simulink model "SF051A_SnsrOffsLrng"  (R2013b)
settings: Solver=FixedStepDiscrete  SolverMode=SingleTasking  StartTime=0.0  StopTime=1  FixedStep=0.002  RelTol=1e-3
undefined symbols (not defined in the file): ARCHGLBPRM_10MILLISEC_SEC_F32, ARCHGLBPRM_2MILLISEC_SEC_F32, ARCHGLBPRM_2PI_ULS_F32, ARCHGLBPRM_FLOATZEROTHD_ULS_F32, ARCHGLBPRM_PIOVER180_ULS_F32, CNV100MICROSECTOMILLISEC_MILLISECPERCNT_F32, CNV100MICROSECTOSEC_SECPERCNT_F32, COVRAMTRXNIT_ULS_F32, HWAUTHYTHD_ULS_F32, HWTQLRNGSTSLRND_CNT_U08, HWTQLRNGSTSNEGOFFS_CNT_U08, HWTQLRNGSTSNOTLRND_CNT_U08, HWTQLRNGSTSPOSOFFS_CNT_U08, HWTQLRNGSTSZEROOFFS_CNT_U08, HWTQLRNGTMRHILIM_SEC_F32, IDYMTRX_ULS_F32, IVS10MS_ULSPERSEC_F32, LRNGFILTICON_ULS_F32, NvmGetErrSts1, ONE_ULS_F32, SnsrOffsLrnd, SnsrOffsLrngFctEna, SnsrOffsLrngHwAgLrngDrvgDstThd, SnsrOffsLrngHwAgLrngEna, SnsrOffsLrngHwAgLrngHwVelThd, SnsrOffsLrngHwAgLrngSysTqThd, SnsrOffsLrngHwAgLrngSysTqThdMed, SnsrOffsLrngHwAgLrngSysTqThdTrustd, SnsrOffsLrngHwAgLrngSysTqThdWide, SnsrOffsLrngHwAgLrngTi, SnsrOffsLrngHwAgLrngVehSpdThd, SnsrOffsLrngHwAgLrngYawOffsDbnd, SnsrOffsLrngHwAgLrngYawRateThd, SnsrOffsLrngHwAgOffsLim, SnsrOffsLrngHwTqLrngEna, SnsrOffsLrngHwTqLrngEnaTiThd, SnsrOffsLrngHwTqLrngHwAgDbnd, SnsrOffsLrngHwTqLrngHwAgThd, SnsrOffsLrngHwTqLrngHwTqThd, SnsrOffsLrngHwTqLrngHwTqZeroOffsThd, SnsrOffsLrngHwTqLrngHwVelThd, SnsrOffsLrngHwTqLrngMeasTi, SnsrOffsLrngHwTqLrngMeasTiScar, SnsrOffsLrngHwTqLrngSampleImbThd1, SnsrOffsLrngHwTqLrngSampleImbThd2, SnsrOffsLrngHwTqLrngSampleThd1, SnsrOffsLrngHwTqLrngSampleThd2, SnsrOffsLrngHwTqLrngTiWghtCoeff, SnsrOffsLrngHwTqLrngVehSpdThd, SnsrOffsLrngHwTqOffsLim, SnsrOffsLrngSampleCntForHwTqLrngRst, SnsrOffsLrngTqInpDetnPwrEstimnThd, SnsrOffsLrngTqInpDetnSinGenrAmp, SnsrOffsLrngTqInpDetnSinGenrFrq, SnsrOffsLrngTqInpDetnStg1FilGain, SnsrOffsLrngTqInpDetnStg1WinSize, SnsrOffsLrngTqInpDetnStg2FilGainCen, SnsrOffsLrngTqInpDetnStg2FilGainDwn, SnsrOffsLrngTqInpDetnStg2FilGainUp, SnsrOffsLrngTqInpDetnStg2WinSize ... (+15)
libraries: Fil x34, FixdToFloat x17, FloatToFixd x16, NxtrLim x15, simulink x12, NxtrAbslt x12, NxtrNvM x8, NxtrMin x5, NxtrMath x3
(part 8 of 11)

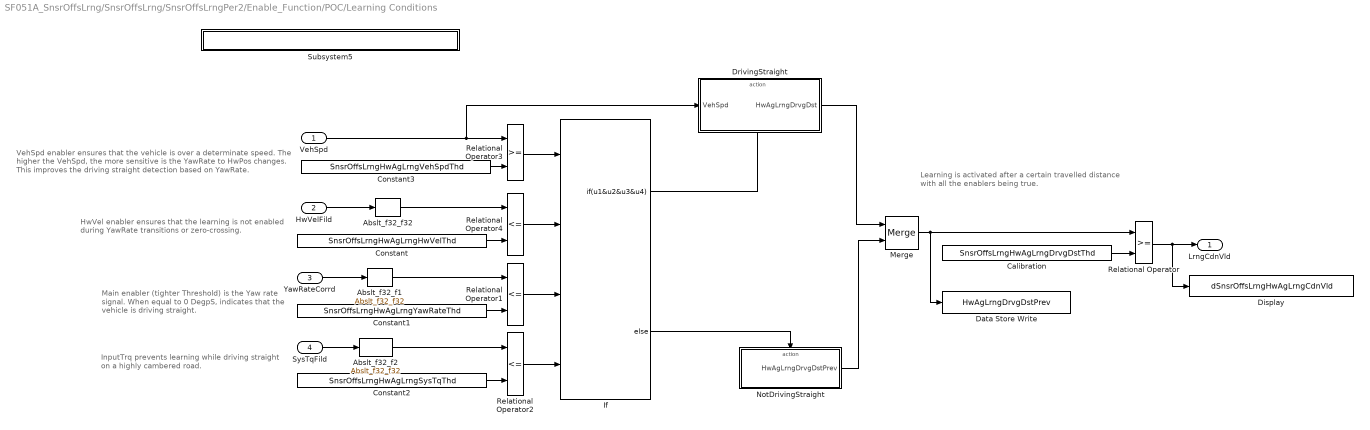
== system SF051A_SnsrOffsLrng/SnsrOffsLrng/SnsrOffsLrngPer2/Enable_Function/POC/Learning Conditions ==
  note: Learning is activated after a certain travelled distance
      |  with all the enablers being true.
  note: InputTrq prevents learning while driving straight
      | on a highly cambered road.
  note: HwVel enabler ensures that the learning is not enabled
      | during YawRate transitions or zero-crossing.
  note: VehSpd enabler ensures that the vehicle is over a determinate speed.
      | The higher the VehSpd, the more sensitive is the YawRate to HwPos
      | changes. This improves the driving straight detection based on YawRate.
  note: Main enabler (tighter Threshold) is the Yaw rate
      | signal. When equal to 0 DegpS, indicates that
      | the vehicle is driving straight.
  VehSpd : Inport  RequirementInfo={'linktype_rmi_doors' '0000babd (/E-STEER Core/SubSystem Specifications/Application Functions/SF051A Sensor Offset Learning)' '#SF051A_125' 'true' 'REQ:SF051A_125' '' } %GIDa_8f59ea37_a6d2_43e8_9752_10147a2ef345
  HwVelFild : Inport  RequirementInfo={'linktype_rmi_doors' '0000babd (/E-STEER Core/SubSystem Specifications/Application Functions/SF051A Sensor Offset Learning)' '#SF051A_125' 'true' 'REQ:SF051A_125' '' } %GIDa_b4c3f45d_537f_4ddb_98c2_1cbec19599c7  Port=2
  YawRateCorrd : Inport  RequirementInfo={'linktype_rmi_doors' '0000babd (/E-STEER Core/SubSystem Specifications/Application Functions/SF051A Sensor Offset Learning)' '#SF051A_125' 'true' 'REQ:SF051A_125' '' } %GIDa_f2d4e035_e9df_4867_bc0f_7342acf6aef2  Port=3
  SysTqFild : Inport  RequirementInfo={'linktype_rmi_doors' '0000babd (/E-STEER Core/SubSystem Specifications/Application Functions/SF051A Sensor Offset Learning)' '#SF051A_125' 'true' 'REQ:SF051A_125' '' } %GIDa_89d517e6_3be2_4d40_b33c_782ff70a0841  Port=4
  Abslt_f32_f1 : NxtrAbslt/Abslt_f32_f32  RequirementInfo={'linktype_rmi_doors' '0000babd (/E-STEER Core/SubSystem Specifications/Application Functions/SF051A Sensor Offset Learning)' '#SF051A_125' 'true' 'REQ:SF051A_125' '' } %GIDa_4a9ff294_23c2_4635_9f2d_79eead891ad6  SFunctionSpec=single y1 = Abslt_f32_f32(single u1)
      settings: AttributesFormatString=%<Name>
  Abslt_f32_f2 : NxtrAbslt/Abslt_f32_f32  RequirementInfo={'linktype_rmi_doors' '0000babd (/E-STEER Core/SubSystem Specifications/Application Functions/SF051A Sensor Offset Learning)' '#SF051A_125' 'true' 'REQ:SF051A_125' '' } %GIDa_bfc6113a_71b3_4014_a79c_4dae946b5258  SFunctionSpec=single y1 = Abslt_f32_f32(single u1)
      settings: AttributesFormatString=%<Name>
  Abslt_f32_f32 : NxtrAbslt/Abslt_f32_f32  RequirementInfo={'linktype_rmi_doors' '0000babd (/E-STEER Core/SubSystem Specifications/Application Functions/SF051A Sensor Offset Learning)' '#SF051A_125' 'true' 'REQ:SF051A_125' '' } %GIDa_d2113858_1e63_4f18_8ebd_0dfc37da8a17  SFunctionSpec=single y1 = Abslt_f32_f32(single u1)
      settings: AttributesFormatString=%<Name>
  Calibration : Constant  RequirementInfo={'linktype_rmi_doors' '0000babd (/E-STEER Core/SubSystem Specifications/Application Functions/SF051A Sensor Offset Learning)' '#SF051A_125' 'true' 'REQ:SF051A_125' '' } %GIDa_a930c023_3647_4bfe_81cc_9ffe63be677e  Value=SnsrOffsLrngHwAgLrngDrvgDstThd  OutDataTypeStr=single
  Constant : Constant  RequirementInfo={'linktype_rmi_doors' '0000babd (/E-STEER Core/SubSystem Specifications/Application Functions/SF051A Sensor Offset Learning)' '#SF051A_125' 'true' 'REQ:SF051A_125' '' } %GIDa_13ca1097_74d2_4314_ac4c_82655165c3ac  Value=SnsrOffsLrngHwAgLrngHwVelThd
  Constant1 : Constant  RequirementInfo={'linktype_rmi_doors' '0000babd (/E-STEER Core/SubSystem Specifications/Application Functions/SF051A Sensor Offset Learning)' '#SF051A_125' 'true' 'REQ:SF051A_125' '' } %GIDa_f59d0f18_d8e0_4a0d_94a2_c992328d5f5a  Value=SnsrOffsLrngHwAgLrngYawRateThd
  Constant2 : Constant  RequirementInfo={'linktype_rmi_doors' '0000babd (/E-STEER Core/SubSystem Specifications/Application Functions/SF051A Sensor Offset Learning)' '#SF051A_125' 'true' 'REQ:SF051A_125' '' } %GIDa_97889c00_0b86_483b_8ac6_8be83d1b4c7e  Value=SnsrOffsLrngHwAgLrngSysTqThd
  Constant3 : Constant  RequirementInfo={'linktype_rmi_doors' '0000babd (/E-STEER Core/SubSystem Specifications/Application Functions/SF051A Sensor Offset Learning)' '#SF051A_125' 'true' 'REQ:SF051A_125' '' } %GIDa_891f1f78_3923_46ac_86af_9c596d3c2421  Value=SnsrOffsLrngHwAgLrngVehSpdThd
  Data Store Write : DataStoreWrite  RequirementInfo={'linktype_rmi_doors' '0000babd (/E-STEER Core/SubSystem Specifications/Application Functions/SF051A Sensor Offset Learning)' '#SF051A_125' 'true' 'REQ:SF051A_125' '' } %GIDa_aa42ae09_446c_4add_b848_b1660a3a4485  DataStoreName=HwAgLrngDrvgDstPrev
  Display : DataStoreWrite  DataStoreName=dSnsrOffsLrngHwAgLrngCdnVld
  DrivingStraight : Subsystem  RequirementInfo={'linktype_rmi_doors' '0000babd (/E-STEER Core/SubSystem Specifications/Application Functions/SF051A Sensor Offset Learning)' '#SF051A_125' 'true' 'REQ:SF051A_125' '' } %GIDa_cc37c45b_3205_4a2a_b2ac_e002ec0e3efb  TreatAsAtomicUnit=on
  If : If  RequirementInfo={'linktype_rmi_doors' '0000babd (/E-STEER Core/SubSystem Specifications/Application Functions/SF051A Sensor Offset Learning)' '#SF051A_125' 'true' 'REQ:SF051A_125' '' } %GIDa_ada5f7e2_fce2_40ad_8932_f71606710b58  NumInputs=4  IfExpression=u1&u2&u3&u4
  Merge : Merge  RequirementInfo={'linktype_rmi_doors' '0000babd (/E-STEER Core/SubSystem Specifications/Application Functions/SF051A Sensor Offset Learning)' '#SF051A_125' 'true' 'REQ:SF051A_125' '' } %GIDa_d84796a1_a26e_43c5_9d0e_55146953274b
  NotDrivingStraight : Subsystem  RequirementInfo={'linktype_rmi_doors' '0000babd (/E-STEER Core/SubSystem Specifications/Application Functions/SF051A Sensor Offset Learning)' '#SF051A_125' 'true' 'REQ:SF051A_125' '' } %GIDa_0603d790_b5f5_4a89_b992_b3578dd6ccf7  TreatAsAtomicUnit=on
  Relational Operator : RelationalOperator  RequirementInfo={'linktype_rmi_doors' '0000babd (/E-STEER Core/SubSystem Specifications/Application Functions/SF051A Sensor Offset Learning)' '#SF051A_125' 'true' 'REQ:SF051A_125' '' } %GIDa_f6c4f543_bc79_4284_beb0_7307c18ad0b4  OutDataTypeStr=boolean
  Relational Operator1 : RelationalOperator  RequirementInfo={'linktype_rmi_doors' '0000babd (/E-STEER Core/SubSystem Specifications/Application Functions/SF051A Sensor Offset Learning)' '#SF051A_125' 'true' 'REQ:SF051A_125' '' } %GIDa_6196e2d7_d842_4412_b387_3769f28bfdab  Operator=<=  OutDataTypeStr=boolean
  Relational Operator2 : RelationalOperator  RequirementInfo={'linktype_rmi_doors' '0000babd (/E-STEER Core/SubSystem Specifications/Application Functions/SF051A Sensor Offset Learning)' '#SF051A_125' 'true' 'REQ:SF051A_125' '' } %GIDa_70a60178_7c67_4179_9a47_94853d13d4d4  Operator=<=  OutDataTypeStr=boolean
  Relational Operator3 : RelationalOperator  RequirementInfo={'linktype_rmi_doors' '0000babd (/E-STEER Core/SubSystem Specifications/Application Functions/SF051A Sensor Offset Learning)' '#SF051A_125' 'true' 'REQ:SF051A_125' '' } %GIDa_022c8ef0_d08f_4bf0_939e_a4515a84757a  OutDataTypeStr=boolean
  Relational Operator4 : RelationalOperator  RequirementInfo={'linktype_rmi_doors' '0000babd (/E-STEER Core/SubSystem Specifications/Application Functions/SF051A Sensor Offset Learning)' '#SF051A_125' 'true' 'REQ:SF051A_125' '' } %GIDa_2be8b1bd_9967_4fbe_97b2_b4364b67bd3a  Operator=<=  OutDataTypeStr=boolean
  Subsystem5 : Subsystem  Description=|  mask(Copyright Information){none=on}
      | Copyright info block.                                               
      |                                                                     
      | Place copyright information at the top of every subsystem in design.
      mask prompts: none "No parameters"
      mask help: Place copyright information at the top of every subsystem in design.
      mask Display:
      | NxtrConf = 'Nexteer Confidential';
      | 
      | sys = bdroot; %handle for the current model ("system")
      | first = get_param(sys,'Created');
      | first = first(end-3:end);  %year is last four digits
      | 
      | last = get_param(sys,'LastModifiedDate');
      | if isempty(last)
      |     last = datestr(now,'yyyy');
      | else
      |     last = last(end-3:end);
      | end
      | 
      | if strcmp(first,last)
      |     fprintf('%s -- Copyright %s Nexteer',NxtrConf,first)
      | else
      |     fprintf('%s -- %s%s- %s Nexteer',NxtrConf,char(169),first,last)
      | end
  LrngCdnVld : Outport
  wires:
  Relational Operator3/1 -> If/1
  HwVelFild/1 -> Abslt_f32_f32/1
  Relational Operator1/1 -> If/3
  Relational Operator4/1 -> If/2
  Abslt_f32_f32/1 -> Relational Operator4/1
  SysTqFild/1 -> Abslt_f32_f2/1
  Relational Operator2/1 -> If/4
  Abslt_f32_f2/1 -> Relational Operator2/1
  Abslt_f32_f1/1 -> Relational Operator1/1
  YawRateCorrd/1 -> Abslt_f32_f1/1
  Constant/1 -> Relational Operator4/2
  Constant1/1 -> Relational Operator1/2
  Constant2/1 -> Relational Operator2/2
  Constant3/1 -> Relational Operator3/2
  If/1 -> DrivingStraight/Action
  If/2 -> NotDrivingStraight/Action
  DrivingStraight/1(HwAgLrngDrvgDst) -> Merge/1
  NotDrivingStraight/1(HwAgLrngDrvgDstPrev) -> Merge/2
  Merge/1 -> Relational Operator/1, Data Store Write/1
  Calibration/1 -> Relational Operator/2
  Relational Operator/1 -> Display/1, LrngCdnVld/1
  VehSpd/1 -> DrivingStraight/1(VehSpd), Relational Operator3/1

== system SF051A_SnsrOffsLrng/SnsrOffsLrng/SnsrOffsLrngPer2/Enable_Function/POC/Reset_HwAg_Learning ==
  note: Suggest coding as inline local function: void Reset_HwAg_Learning()
  note: Set HwAg Offlset learning filter back to the last good learned value written to NVM Ram.
      | Set elapsed learning time back to zero.
  note: Reset timer
  note: Reset filters
  Action Port : ActionPort  ActionType=then
  Constant : Constant  Value=ZERO_ULS_F32  OutDataTypeStr=single
      settings: AttributesFormatString=%<OutDataTypeStr>
  Filter SV : DataStoreWrite  DataStoreName=HwAgLrngFil1  DataStoreElements=HwAgLrngFil1.FilSt
  Filter SV1 : DataStoreWrite  DataStoreName=HwAgLrngFil2  DataStoreElements=HwAgLrngFil2.FilSt
  FixdToFloat_f32_s16 : FixdToFloat/FixdToFloat_f32_s16  Param1=10
  NVMRam_Read : DataStoreRead  DataStoreName=SnsrOffsLrnd  DataStoreElements=SnsrOffsLrnd.YawRateOffs
  Read NVM Ram : DataStoreRead  DataStoreName=SnsrOffsLrnd  DataStoreElements=SnsrOffsLrnd.HwAgOffs
  Subsystem5 : Subsystem  Description=|  mask(Copyright Information){none=on}
      | Copyright info block.                                               
      |                                                                     
      | Place copyright information at the top of every subsystem in design.
      mask prompts: none "No parameters"
      mask help: Place copyright information at the top of every subsystem in design.
      mask Display:
      | NxtrConf = 'Nexteer Confidential';
      | 
      | sys = bdroot; %handle for the current model ("system")
      | first = get_param(sys,'Created');
      | first = first(end-3:end);  %year is last four digits
      | 
      | last = get_param(sys,'LastModifiedDate');
      | if isempty(last)
      |     last = datestr(now,'yyyy');
      | else
      |     last = last(end-3:end);
      | end
      | 
      | if strcmp(first,last)
      |     fprintf('%s -- Copyright %s Nexteer',NxtrConf,first)
      | else
      |     fprintf('%s -- %s%s- %s Nexteer',NxtrConf,char(169),first,last)
      | end
  Update Reference : DataStoreWrite  DataStoreName=SnsrOffsLrnd  DataStoreElements=SnsrOffsLrnd.HwAgLrngYawOffsRef
  Write NVM Ram : DataStoreWrite  DataStoreName=SnsrOffsLrnd  DataStoreElements=SnsrOffsLrnd.HwAgLrndTi
  wires:
  Constant/1 -> Write NVM Ram/1
  Read NVM Ram/1 -> FixdToFloat_f32_s16/1
  NVMRam_Read/1 -> Update Reference/1
  FixdToFloat_f32_s16/1 -> Filter SV1/1, Filter SV/1

== system SF051A_SnsrOffsLrng/SnsrOffsLrng/SnsrOffsLrngPer2/Enable_Function/POC/Subsystem5 ==

== system SF051A_SnsrOffsLrng/SnsrOffsLrng/SnsrOffsLrngPer2/Enable_Function/SOaC_HierarchyManager/POCEnabler ==
  CmnSigVld : Inport  RequirementInfo={'linktype_rmi_doors' '0000babd (/E-STEER Core/SubSystem Specifications/Application Functions/SF051A Sensor Offset Learning)' '#SF051A_135' 'true' 'REQ:SF051A_135' '' } %GIDa_a3a90e4b_a515_4369_8278_0f9e775efabb
  VehYawRateVld : Inport  RequirementInfo={'linktype_rmi_doors' '0000babd (/E-STEER Core/SubSystem Specifications/Application Functions/SF051A Sensor Offset Learning)' '#SF051A_135' 'true' 'REQ:SF051A_135' '' } %GIDa_046d27fa_e356_4762_86a1_0902f3c2ade4  Port=2
  YawRateOffsFrsh : Inport  RequirementInfo={'linktype_rmi_doors' '0000babd (/E-STEER Core/SubSystem Specifications/Application Functions/SF051A Sensor Offset Learning)' '#SF051A_135' 'true' 'REQ:SF051A_135' '' } %GIDa_03f8236f_a4d8_4504_bef2_73d121deb598  Port=3
  Constant1 : Constant  RequirementInfo={'linktype_rmi_doors' '0000babd (/E-STEER Core/SubSystem Specifications/Application Functions/SF051A Sensor Offset Learning)' '#SF051A_136' 'true' 'REQ:SF051A_136' '' ; 'linktype_rmi_doors' '0000babd (/E-STEER Core/SubSystem Specifications/Application Functions/SF051A Sensor Offset Learning)' '#SF051A_135' 'true' 'REQ:SF051A_135' '' } %GIDa_886d2d83_0f18_47ff_afe5_95719c677a16  Value=SnsrOffsLrngHwAgLrngEna
  Display : DataStoreWrite  DataStoreName=dSnsrOffsLrngHwAgLrngEna
  Logical Operator : Logic  RequirementInfo={'linktype_rmi_doors' '0000babd (/E-STEER Core/SubSystem Specifications/Application Functions/SF051A Sensor Offset Learning)' '#SF051A_135' 'true' 'REQ:SF051A_135' '' ; 'linktype_rmi_doors' '0000babd (/E-STEER Core/SubSystem Specifications/Application Functions/SF051A Sensor Offset Learning)' '#SF051A_136' 'true' 'REQ:SF051A_136' '' } %GIDa_e1d92644_86b9_417b_bb7c_d622c0b2c40b  Inputs=5  AllPortsSameDT=off  OutDataTypeStr=boolean
  NvmRam : DataStoreRead  RequirementInfo={'linktype_rmi_doors' '0000babd (/E-STEER Core/SubSystem Specifications/Application Functions/SF051A Sensor Offset Learning)' '#SF051A_135' 'true' 'REQ:SF051A_135' '' } %GIDa_d64055b6_ad18_4625_99bc_bc222697d718  DataStoreName=SnsrOffsLrnd  DataStoreElements=SnsrOffsLrnd.YawRateOffsVld
  Subsystem5 : Subsystem  Description=|  mask(Copyright Information){none=on}
      | Copyright info block.                                               
      |                                                                     
      | Place copyright information at the top of every subsystem in design.
      mask prompts: none "No parameters"
      mask help: Place copyright information at the top of every subsystem in design.
      mask Display:
      | NxtrConf = 'Nexteer Confidential';
      | 
      | sys = bdroot; %handle for the current model ("system")
      | first = get_param(sys,'Created');
      | first = first(end-3:end);  %year is last four digits
      | 
      | last = get_param(sys,'LastModifiedDate');
      | if isempty(last)
      |     last = datestr(now,'yyyy');
      | else
      |     last = last(end-3:end);
      | end
      | 
      | if strcmp(first,last)
      |     fprintf('%s -- Copyright %s Nexteer',NxtrConf,first)
      | else
      |     fprintf('%s -- %s%s- %s Nexteer',NxtrConf,char(169),first,last)
      | end
  HwAgLrngEna : Outport
  wires:
  Logical Operator/1 -> Display/1, HwAgLrngEna/1
  CmnSigVld/1 -> Logical Operator/2
  Constant1/1 -> Logical Operator/1
  YawRateOffsFrsh/1 -> Logical Operator/4
  NvmRam/1 -> Logical Operator/5
  VehYawRateVld/1 -> Logical Operator/3

== system SF051A_SnsrOffsLrng/SnsrOffsLrng/SnsrOffsLrngPer2/Enable_Function/SOaC_HierarchyManager/POCResetLogic ==
  note: Capture the learned Yaw Rate Offset each time that HwAg learning is reset.  If at any time
      | Yaw Rate Offset changes significantly from the captured reference value, reset the HwAg
      | learning routine.  In other words, a major change in Yaw triggers a re-learn of HwAg.
  Abslt_f32_f32 : NxtrAbslt/Abslt_f32_f32  RequirementInfo={'linktype_rmi_doors' '0000babd (/E-STEER Core/SubSystem Specifications/Application Functions/SF051A Sensor Offset Learning)' '#SF051A_134' 'true' 'REQ:SF051A_134' '' } %GIDa_eb268217_533f_429b_abe3_8ca1827af580  SFunctionSpec=single y1 = Abslt_f32_f32(single u1)
      settings: AttributesFormatString=%<Name>
  Constant : Constant  RequirementInfo={'linktype_rmi_doors' '0000babd (/E-STEER Core/SubSystem Specifications/Application Functions/SF051A Sensor Offset Learning)' '#SF051A_134' 'true' 'REQ:SF051A_134' '' } %GIDa_cb9b8ced_48a1_40df_bd9e_7bf129476d0f  Value=SnsrOffsLrngHwAgLrngYawOffsDbnd
  Data Store Read : DataStoreRead  RequirementInfo={'linktype_rmi_doors' '0000babd (/E-STEER Core/SubSystem Specifications/Application Functions/SF051A Sensor Offset Learning)' '#SF051A_134' 'true' 'REQ:SF051A_134' '' } %GIDa_76c40593_7955_4a5c_86c5_bdfe212e95b7  DataStoreName=SnsrOffsLrnd  DataStoreElements=SnsrOffsLrnd.HwAgLrngYawOffsRef
  Display : DataStoreWrite  DataStoreName=dSnsrOffsLrngHwAgLrngRst
  FixdToFloat_f32_s1 : FixdToFloat/FixdToFloat_f32_s16  RequirementInfo={'linktype_rmi_doors' '0000babd (/E-STEER Core/SubSystem Specifications/Application Functions/SF051A Sensor Offset Learning)' '#SF051A_134' 'true' 'REQ:SF051A_134' '' } %GIDa_6455c289_ed33_4177_b6b5_a172c9b77801  Param1=9
  FixdToFloat_f32_s16 : FixdToFloat/FixdToFloat_f32_s16  RequirementInfo={'linktype_rmi_doors' '0000babd (/E-STEER Core/SubSystem Specifications/Application Functions/SF051A Sensor Offset Learning)' '#SF051A_134' 'true' 'REQ:SF051A_134' '' } %GIDa_7b39a599_1da3_484b_8e4f_9eef5a9ab7b8  Param1=9
  NVMRam_Read : DataStoreRead  RequirementInfo={'linktype_rmi_doors' '0000babd (/E-STEER Core/SubSystem Specifications/Application Functions/SF051A Sensor Offset Learning)' '#SF051A_134' 'true' 'REQ:SF051A_134' '' } %GIDa_7759f917_66ca_4690_a4ef_7d43ee1a0bc2  DataStoreName=SnsrOffsLrnd  DataStoreElements=SnsrOffsLrnd.YawRateOffs
  Relational Operator : RelationalOperator  RequirementInfo={'linktype_rmi_doors' '0000babd (/E-STEER Core/SubSystem Specifications/Application Functions/SF051A Sensor Offset Learning)' '#SF051A_134' 'true' 'REQ:SF051A_134' '' } %GIDa_3c7dc04c_6755_4531_889f_25e567f76468  OutDataTypeStr=boolean
  Subsystem5 : Subsystem  Description=|  mask(Copyright Information){none=on}
      | Copyright info block.                                               
      |                                                                     
      | Place copyright information at the top of every subsystem in design.
      mask prompts: none "No parameters"
      mask help: Place copyright information at the top of every subsystem in design.
      mask Display:
      | NxtrConf = 'Nexteer Confidential';
      | 
      | sys = bdroot; %handle for the current model ("system")
      | first = get_param(sys,'Created');
      | first = first(end-3:end);  %year is last four digits
      | 
      | last = get_param(sys,'LastModifiedDate');
      | if isempty(last)
      |     last = datestr(now,'yyyy');
      | else
      |     last = last(end-3:end);
      | end
      | 
      | if strcmp(first,last)
      |     fprintf('%s -- Copyright %s Nexteer',NxtrConf,first)
      | else
      |     fprintf('%s -- %s%s- %s Nexteer',NxtrConf,char(169),first,last)
      | end
  Subtract : Sum  RequirementInfo={'linktype_rmi_doors' '0000babd (/E-STEER Core/SubSystem Specifications/Application Functions/SF051A Sensor Offset Learning)' '#SF051A_134' 'true' 'REQ:SF051A_134' '' } %GIDa_8b9d9596_8162_48c0_9d38_f3b9f3ab54f1  Inputs=+-
  HwAgLrngRst : Outport
  wires:
  Abslt_f32_f32/1 -> Relational Operator/1
  Subtract/1 -> Abslt_f32_f32/1
  Constant/1 -> Relational Operator/2
  NVMRam_Read/1 -> FixdToFloat_f32_s16/1
  Data Store Read/1 -> FixdToFloat_f32_s1/1
  Relational Operator/1 -> Display/1, HwAgLrngRst/1
  FixdToFloat_f32_s16/1 -> Subtract/1
  FixdToFloat_f32_s1/1 -> Subtract/2

== system SF051A_SnsrOffsLrng/SnsrOffsLrng/SnsrOffsLrngPer2/Enable_Function/SOaC_HierarchyManager/Subsystem5 ==

== system SF051A_SnsrOffsLrng/SnsrOffsLrng/SnsrOffsLrngPer2/Enable_Function/SOaC_HierarchyManager/YOCEnabler ==
  note: YOC is enabled if:
      |   - YOCEnable is true
      |   - InputSIgnals Authority is 1
  CmnSigVld : Inport
  VehYawRateVld : Inport  Port=2
  Constant1 : Constant  RequirementInfo={'linktype_rmi_doors' '0000babd (/E-STEER Core/SubSystem Specifications/Application Functions/SF051A Sensor Offset Learning)' '#SF051A_32' 'true' 'REQ:SF051A_32' '' } %GIDa_be471898_d215_4b61_9c96_ada0f6355517  Value=SnsrOffsLrngYawLrngEna
  Display : DataStoreWrite  DataStoreName=dSnsrOffsLrngYawLrngEna
  Logical Operator : Logic  RequirementInfo={'linktype_rmi_doors' '0000babd (/E-STEER Core/SubSystem Specifications/Application Functions/SF051A Sensor Offset Learning)' '#SF051A_32' 'true' 'REQ:SF051A_32' '' } %GIDa_c6731b2d_5e96_4da6_8262_b10b0921fb99  Inputs=3  AllPortsSameDT=off  OutDataTypeStr=boolean
  Subsystem5 : Subsystem  Description=|  mask(Copyright Information){none=on}
      | Copyright info block.                                               
      |                                                                     
      | Place copyright information at the top of every subsystem in design.
      mask prompts: none "No parameters"
      mask help: Place copyright information at the top of every subsystem in design.
      mask Display:
      | NxtrConf = 'Nexteer Confidential';
      | 
      | sys = bdroot; %handle for the current model ("system")
      | first = get_param(sys,'Created');
      | first = first(end-3:end);  %year is last four digits
      | 
      | last = get_param(sys,'LastModifiedDate');
      | if isempty(last)
      |     last = datestr(now,'yyyy');
      | else
      |     last = last(end-3:end);
      | end
      | 
      | if strcmp(first,last)
      |     fprintf('%s -- Copyright %s Nexteer',NxtrConf,first)
      | else
      |     fprintf('%s -- %s%s- %s Nexteer',NxtrConf,char(169),first,last)
      | end
  YawRateLrngEna : Outport
  wires:
  Constant1/1 -> Logical Operator/1
  CmnSigVld/1 -> Logical Operator/2
  Logical Operator/1 -> Display/1, YawRateLrngEna/1
  VehYawRateVld/1 -> Logical Operator/3

== system SF051A_SnsrOffsLrng/SnsrOffsLrng/SnsrOffsLrngPer2/Enable_Function/YOC/Do nothing ==
  Action Port : ActionPort  ActionType=else
  Subsystem5 : Subsystem  Description=|  mask(Copyright Information){none=on}
      | Copyright info block.                                               
      |                                                                     
      | Place copyright information at the top of every subsystem in design.
      mask prompts: none "No parameters"
      mask help: Place copyright information at the top of every subsystem in design.
      mask Display:
      | NxtrConf = 'Nexteer Confidential';
      | 
      | sys = bdroot; %handle for the current model ("system")
      | first = get_param(sys,'Created');
      | first = first(end-3:end);  %year is last four digits
      | 
      | last = get_param(sys,'LastModifiedDate');
      | if isempty(last)
      |     last = datestr(now,'yyyy');
      | else
      |     last = last(end-3:end);
      | end
      | 
      | if strcmp(first,last)
      |     fprintf('%s -- Copyright %s Nexteer',NxtrConf,first)
      | else
      |     fprintf('%s -- %s%s- %s Nexteer',NxtrConf,char(169),first,last)
      | end

== system SF051A_SnsrOffsLrng/SnsrOffsLrng/SnsrOffsLrngPer2/Enable_Function/YOC/Learn ==
  note: Entrance to this subsystem means that vehicle conditions are good for learning.
      |
      | When leaving factory, or after an external reset, consider the learned offset not valid until the filters have had a tunable length of time to
      | attain good approximation of true offset.  Once the learned offset is deemed valid, the timing constraint is removed so that being parked
      | even for a few seconds may tweak the learned value a bit.
      |
      | Filter continuously, but if the duration is not sufficient, do not update NVM RAM with new value.  Next time conditions are good, the filters
      | will continue from their last values.
  note: Filters are continuously active inside this subsystem.  When
      | not in this subystem, the filter state variables are frozen.
  note: Limit changed to a Min block.
  YawRate : Inport
  Action Port : ActionPort  ActionType=then
  Add : Sum  RequirementInfo={'linktype_rmi_doors' '0000babd (/E-STEER Core/SubSystem Specifications/Application Functions/SF051A Sensor Offset Learning)' '#SF051A_90' 'true' 'REQ:SF051A_90' '' } %GIDa_f07b436d_1106_4fd0_930e_f28a3eb3dbeb
  Constant : Constant  RequirementInfo={'linktype_rmi_doors' '0000babd (/E-STEER Core/SubSystem Specifications/Application Functions/SF051A Sensor Offset Learning)' '#SF051A_93' 'true' 'REQ:SF051A_93' '' } %GIDa_394b4221_be42_4a57_8d0b_59a834239b66  Value=SnsrOffsLrngYawLrngTi
  Constant1 : Constant  RequirementInfo={'linktype_rmi_doors' '0000babd (/E-STEER Core/SubSystem Specifications/Application Functions/SF051A Sensor Offset Learning)' '#SF051A_90' 'true' 'REQ:SF051A_90' '' } %GIDa_2c7cd52d_897c_453e_ac97_2e50719e1535  Value=SnsrOffsLrngYawLrngTi
  Constant2 : Constant  RequirementInfo={'linktype_rmi_doors' '0000babd (/E-STEER Core/SubSystem Specifications/Application Functions/SF051A Sensor Offset Learning)' '#SF051A_90' 'true' 'REQ:SF051A_90' '' } %GIDa_9ba959ec_8787_4e5e_bf59_5b49aec7d530  Value=ARCHGLBPRM_10MILLISEC_SEC_F32
  Data Store Read1 : DataStoreRead  RequirementInfo={'linktype_rmi_doors' '0000babd (/E-STEER Core/SubSystem Specifications/Application Functions/SF051A Sensor Offset Learning)' '#SF051A_90' 'true' 'REQ:SF051A_90' '' } %GIDa_8a94f522_706f_4c34_96a1_0958abef325c  DataStoreName=YawLrngElpdLrngTi
  Data Store Read2 : DataStoreRead  RequirementInfo={'linktype_rmi_doors' '0000babd (/E-STEER Core/SubSystem Specifications/Application Functions/SF051A Sensor Offset Learning)' '#SF051A_107' 'true' 'REQ:SF051A_107' '' } %GIDa_e5d570d4_63e2_441f_9653_8a3e1892128d  DataStoreName=SnsrOffsLrnd  DataStoreElements=SnsrOffsLrnd.YawRateOffsVld
  Data Store Write : DataStoreWrite  RequirementInfo={'linktype_rmi_doors' '0000babd (/E-STEER Core/SubSystem Specifications/Application Functions/SF051A Sensor Offset Learning)' '#SF051A_91' 'true' 'REQ:SF051A_91' '' ; 'linktype_rmi_doors' '0000babd (/E-STEER Core/SubSystem Specifications/Application Functions/SF051A Sensor Offset Learning)' '#SF051A_240' 'true' 'REQ:SF051A_240' '' } %GIDa_b4784234_42bd_4e32_bd30_b08c662a4725  DataStoreName=YawLrngElpdLrngTi
  Do nothing : Subsystem  TreatAsAtomicUnit=on
  Filter For Learning : Subsystem
  If : If  RequirementInfo={'linktype_rmi_doors' '0000babd (/E-STEER Core/SubSystem Specifications/Application Functions/SF051A Sensor Offset Learning)' '#SF051A_107' 'true' 'REQ:SF051A_107' '' } %GIDa_5a864c38_8cd9_4e7a_b628_0403566d2c9a  NumInputs=2  IfExpression=u1 | u2
  Min_f32 : NxtrMin/Min_f32  SFunctionSpec=single y1 = Min_f32(single u1, single u2)
      settings: AttributesFormatString=%<Name>
  Relational Operator : RelationalOperator  RequirementInfo={'linktype_rmi_doors' '0000babd (/E-STEER Core/SubSystem Specifications/Application Functions/SF051A Sensor Offset Learning)' '#SF051A_107' 'true' 'REQ:SF051A_107' '' } %GIDa_09260735_486f_484e_9884_e2f31241b5f4  Operator=>  OutDataTypeStr=boolean
  Subsystem5 : Subsystem  Description=|  mask(Copyright Information){none=on}
      | Copyright info block.                                               
      |                                                                     
      | Place copyright information at the top of every subsystem in design.
      mask prompts: none "No parameters"
      mask help: Place copyright information at the top of every subsystem in design.
      mask Display:
      | NxtrConf = 'Nexteer Confidential';
      | 
      | sys = bdroot; %handle for the current model ("system")
      | first = get_param(sys,'Created');
      | first = first(end-3:end);  %year is last four digits
      | 
      | last = get_param(sys,'LastModifiedDate');
      | if isempty(last)
      |     last = datestr(now,'yyyy');
      | else
      |     last = last(end-3:end);
      | end
      | 
      | if strcmp(first,last)
      |     fprintf('%s -- Copyright %s Nexteer',NxtrConf,first)
      | else
      |     fprintf('%s -- %s%s- %s Nexteer',NxtrConf,char(169),first,last)
      | end
  Update NVM RAM : Subsystem  TreatAsAtomicUnit=on
  wires:
  Add/1 -> Min_f32/1, Relational Operator/1  "ElpsdTi_Sec_T_f32"
  YawRate/1 -> Filter For Learning/1(YawRate)
  Filter For Learning/1(LrndBias) -> Update NVM RAM/1(LrndBias)
  If/1 -> Update NVM RAM/Action
  Data Store Read1/1 -> Add/1
  Constant2/1 -> Add/2
  Min_f32/1 -> Data Store Write/1
  Data Store Read2/1 -> If/1
  Constant/1 -> Relational Operator/2
  Relational Operator/1 -> If/2
  If/2 -> Do nothing/Action
  Constant1/1 -> Min_f32/2

== system SF051A_SnsrOffsLrng/SnsrOffsLrng/SnsrOffsLrngPer2/Enable_Function/YOC/Learning Conditions ==
  note: VehSpd = 0 kph is taken as the reference condition
      | for YawRate = 0 DegperS
  note: HwPos <= Threshold is used to prevent learning
      | at very low VehSpd. Vehicle speed sensors are not reliable
      | at values close to 0 kph. If the Hand wheel is in a position near
      | on center, the YawRate signal will not have a big value when the vehicle
      | starts or stops moving.
  note: YawRate <= Threshold  AND YawRate_Gradient <= Threshold
      | are used to prevent learning when the vehicle is located stopped on
      | a moving platform (e.g. Japanish parkings, ferries)
  VehSpd : Inport
  HwAg : Inport  Port=2
  YawA : Inport  Port=3
  YawRateFild : Inport  Port=4  OutDataTypeStr=single
  Abslt_f32_f1 : NxtrAbslt/Abslt_f32_f32  SFunctionSpec=single y1 = Abslt_f32_f32(single u1)
      settings: AttributesFormatString=%<Name>
  Abslt_f32_f2 : NxtrAbslt/Abslt_f32_f32  SFunctionSpec=single y1 = Abslt_f32_f32(single u1)
      settings: AttributesFormatString=%<Name>
  Abslt_f32_f32 : NxtrAbslt/Abslt_f32_f32  SFunctionSpec=single y1 = Abslt_f32_f32(single u1)
      settings: AttributesFormatString=%<Name>
  Add : Sum
  Constant : Constant  Value=SnsrOffsLrngYawLrngHwAgThd
  Constant1 : Constant  Value=SnsrOffsLrngYawLrngYawAThd
  Constant2 : Constant  Value=SnsrOffsLrngYawRateOffsLim
  Constant3 : Constant  Value=YAWRATENOISE_VEHDEGPERSEC_F32
  Display : DataStoreWrite  DataStoreName=dSnsrOffsLrngYawLrngCdnVld
  Float Zero : Constant  Value=ARCHGLBPRM_FLOATZEROTHD_ULS_F32
  Logical Operator : Logic  Inputs=4  AllPortsSameDT=off  OutDataTypeStr=boolean
  Relational Operator{1..4} (4 alike) : RelationalOperator  Operator=<=  OutDataTypeStr=boolean
  Subsystem5 : Subsystem  Description=|  mask(Copyright Information){none=on}
      | Copyright info block.                                               
      |                                                                     
      | Place copyright information at the top of every subsystem in design.
      mask prompts: none "No parameters"
      mask help: Place copyright information at the top of every subsystem in design.
      mask Display:
      | NxtrConf = 'Nexteer Confidential';
      | 
      | sys = bdroot; %handle for the current model ("system")
      | first = get_param(sys,'Created');
      | first = first(end-3:end);  %year is last four digits
      | 
      | last = get_param(sys,'LastModifiedDate');
      | if isempty(last)
      |     last = datestr(now,'yyyy');
      | else
      |     last = last(end-3:end);
      | end
      | 
      | if strcmp(first,last)
      |     fprintf('%s -- Copyright %s Nexteer',NxtrConf,first)
      | else
      |     fprintf('%s -- %s%s- %s Nexteer',NxtrConf,char(169),first,last)
      | end
  LrngCdnVld : Outport
  wires:
  VehSpd/1 -> Relational Operator1/1
  HwAg/1 -> Abslt_f32_f32/1
  Abslt_f32_f32/1 -> Relational Operator4/1
  Relational Operator1/1 -> Logical Operator/1
  Relational Operator4/1 -> Logical Operator/2
  Constant/1 -> Relational Operator4/2
  Float Zero/1 -> Relational Operator1/2
  Abslt_f32_f2/1 -> Relational Operator3/1
  YawA/1 -> Abslt_f32_f2/1
  YawRateFild/1 -> Abslt_f32_f1/1
  Abslt_f32_f1/1 -> Relational Operator2/1
  Constant1/1 -> Relational Operator3/2
  Add/1 -> Relational Operator2/2
  Relational Operator2/1 -> Logical Operator/3
  Relational Operator3/1 -> Logical Operator/4
  Constant3/1 -> Add/1
  Constant2/1 -> Add/2
  Logical Operator/1 -> Display/1, LrngCdnVld/1

== system SF051A_SnsrOffsLrng/SnsrOffsLrng/SnsrOffsLrngPer2/Enable_Function/YOC/Subsystem5 ==

== system SF051A_SnsrOffsLrng/SnsrOffsLrng/SnsrOffsLrngPer1/EnableLearning/EnablingConditions/CheckLastMeasHwPos/FalseOut_KeepRef ==
  Action Port : ActionPort  ActionType=else
  Constant : Constant  Value=false  OutDataTypeStr=boolean
      settings: AttributesFormatString=%<OutDataTypeStr>
  Subsystem5 : Subsystem  Description=|  mask(Copyright Information){none=on}
      | Copyright info block.                                               
      |                                                                     
      | Place copyright information at the top of every subsystem in design.
      mask prompts: none "No parameters"
      mask help: Place copyright information at the top of every subsystem in design.
      mask Display:
      | NxtrConf = 'Nexteer Confidential';
      | 
      | sys = bdroot; %handle for the current model ("system")
      | first = get_param(sys,'Created');
      | first = first(end-3:end);  %year is last four digits
      | 
      | last = get_param(sys,'LastModifiedDate');
      | if isempty(last)
      |     last = datestr(now,'yyyy');
      | else
      |     last = last(end-3:end);
      | end
      | 
      | if strcmp(first,last)
      |     fprintf('%s -- Copyright %s Nexteer',NxtrConf,first)
      | else
      |     fprintf('%s -- %s%s- %s Nexteer',NxtrConf,char(169),first,last)
      | end
  HwAgMoved : Outport
  wires:
  Constant/1 -> HwAgMoved/1

== system SF051A_SnsrOffsLrng/SnsrOffsLrng/SnsrOffsLrngPer1/EnableLearning/EnablingConditions/CheckLastMeasHwPos/Subsystem5 ==

== system SF051A_SnsrOffsLrng/SnsrOffsLrng/SnsrOffsLrngPer1/EnableLearning/EnablingConditions/CheckLastMeasHwPos/TrueOut_ResetRef ==
  Action Port : ActionPort  ActionType=then
  Constant : Constant  Value=true  OutDataTypeStr=boolean
      settings: AttributesFormatString=%<OutDataTypeStr>
  Constant1 : Constant  Value=SYSGLBPRM_HWAGHILIM_HWDEG_F32  OutDataTypeStr=single
  FloatToFixd_s16_f32 : FloatToFixd/FloatToFixd_s16_f32  Param1=4
  NVM write : DataStoreWrite  DataStoreName=SnsrOffsLrnd  DataStoreElements=SnsrOffsLrnd.HwTqLrngHwAgRef
  Subsystem5 : Subsystem  Description=|  mask(Copyright Information){none=on}
      | Copyright info block.                                               
      |                                                                     
      | Place copyright information at the top of every subsystem in design.
      mask prompts: none "No parameters"
      mask help: Place copyright information at the top of every subsystem in design.
      mask Display:
      | NxtrConf = 'Nexteer Confidential';
      | 
      | sys = bdroot; %handle for the current model ("system")
      | first = get_param(sys,'Created');
      | first = first(end-3:end);  %year is last four digits
      | 
      | last = get_param(sys,'LastModifiedDate');
      | if isempty(last)
      |     last = datestr(now,'yyyy');
      | else
      |     last = last(end-3:end);
      | end
      | 
      | if strcmp(first,last)
      |     fprintf('%s -- Copyright %s Nexteer',NxtrConf,first)
      | else
      |     fprintf('%s -- %s%s- %s Nexteer',NxtrConf,char(169),first,last)
      | end
  HwAgMoved : Outport
  wires:
  Constant/1 -> HwAgMoved/1
  Constant1/1 -> FloatToFixd_s16_f32/1
  FloatToFixd_s16_f32/1 -> NVM write/1

== system SF051A_SnsrOffsLrng/SnsrOffsLrng/SnsrOffsLrngPer1/EnableLearning/Eval_Time/GetTiSpan100MicroSec32bit/CopyRight2 ==

== system SF051A_SnsrOffsLrng/SnsrOffsLrng/SnsrOffsLrngPer1/EnableLearning/Eval_Time/GetTiSpan100MicroSec32bit/No wrapping ==
  new : Inport
  ref : Inport  Port=2
  Action Port : ActionPort  ActionType=then
  CopyRight2 : Subsystem  Description=|  mask(Copyright Information){none=on}
      | Copyright info block.                                               
      |                                                                     
      | Place copyright information at the top of every subsystem in design.
      mask prompts: none "No parameters"
      mask help: Place copyright information at the top of every subsystem in design.
      mask Display:
      | NxtrConf = 'Nexteer Confidential';
      | 
      | sys = bdroot; %handle for the current model ("system")
      | first = get_param(sys,'Created');
      | if(isempty(first))
      |     first = datestr(now,'yyyy');
      | else
      |     first = first(end-3:end);  %year is last four digits
      | end
      | 
      | last = get_param(sys,'LastModifiedDate');
      | if isempty(last)
      |     last = datestr(now,'yyyy');
      | else
      |     last = last(end-3:end);
      | end
      | 
      | if strcmp(first,last)
      |     fprintf('%s -- Copyright %s Nexteer',NxtrConf,first)
      | else
      |     fprintf('%s -- %s%s- %s Nexteer',NxtrConf,char(169),first,last)
      | end
  Subtract1 : Sum  Inputs=+-
  Out1 : Outport
  wires:
  ref/1 -> Subtract1/2
  new/1 -> Subtract1/1
  Subtract1/1 -> Out1/1

== system SF051A_SnsrOffsLrng/SnsrOffsLrng/SnsrOffsLrngPer1/EnableLearning/Eval_Time/GetTiSpan100MicroSec32bit/Wrapping ==
  new : Inport
  ref : Inport  Port=2
  Action Port : ActionPort  ActionType=else
  CopyRight2 : Subsystem  Description=|  mask(Copyright Information){none=on}
      | Copyright info block.                                               
      |                                                                     
      | Place copyright information at the top of every subsystem in design.
      mask prompts: none "No parameters"
      mask help: Place copyright information at the top of every subsystem in design.
      mask Display:
      | NxtrConf = 'Nexteer Confidential';
      | 
      | sys = bdroot; %handle for the current model ("system")
      | first = get_param(sys,'Created');
      | if(isempty(first))
      |     first = datestr(now,'yyyy');
      | else
      |     first = first(end-3:end);  %year is last four digits
      | end
      | 
      | last = get_param(sys,'LastModifiedDate');
      | if isempty(last)
      |     last = datestr(now,'yyyy');
      | else
      |     last = last(end-3:end);
      | end
      | 
      | if strcmp(first,last)
      |     fprintf('%s -- Copyright %s Nexteer',NxtrConf,first)
      | else
      |     fprintf('%s -- %s%s- %s Nexteer',NxtrConf,char(169),first,last)
      | end
  Max Counts : Constant  Value=2^32-1  OutDataTypeStr=uint32
  Subtract1 : Sum  Inputs=+-+
  Out1 : Outport
  wires:
  new/1 -> Subtract1/3
  ref/1 -> Subtract1/2
  Max Counts/1 -> Subtract1/1
  Subtract1/1 -> Out1/1

== system SF051A_SnsrOffsLrng/SnsrOffsLrng/SnsrOffsLrngPer1/EnableLearning/False_Reset/GetRefTmr100MicroSec32bit/CopyRight2 ==

== system SF051A_SnsrOffsLrng/SnsrOffsLrng/SnsrOffsLrngPer1/EnableLearning/Perform_TqInpDetn/Do nothing/Subsystem5 ==

== system SF051A_SnsrOffsLrng/SnsrOffsLrng/SnsrOffsLrngPer1/EnableLearning/Perform_TqInpDetn/ElapsedTime/Subsystem5 ==

== system SF051A_SnsrOffsLrng/SnsrOffsLrng/SnsrOffsLrngPer1/EnableLearning/Perform_TqInpDetn/Enable_PreProcessing/False_Hold ==
  Action Port : ActionPort  ActionType=else
  Constant : Constant  Value=false  OutDataTypeStr=boolean
      settings: AttributesFormatString=%<OutDataTypeStr>
  Previous_Value : DataStoreRead  DataStoreName=HwTqLrngTqInpPrsnt
  Subsystem5 : Subsystem  Description=|  mask(Copyright Information){none=on}
      | Copyright info block.                                               
      |                                                                     
      | Place copyright information at the top of every subsystem in design.
      mask prompts: none "No parameters"
      mask help: Place copyright information at the top of every subsystem in design.
      mask Display:
      | NxtrConf = 'Nexteer Confidential';
      | 
      | sys = bdroot; %handle for the current model ("system")
      | first = get_param(sys,'Created');
      | first = first(end-3:end);  %year is last four digits
      | 
      | last = get_param(sys,'LastModifiedDate');
      | if isempty(last)
      |     last = datestr(now,'yyyy');
      | else
      |     last = last(end-3:end);
      | end
      | 
      | if strcmp(first,last)
      |     fprintf('%s -- Copyright %s Nexteer',NxtrConf,first)
      | else
      |     fprintf('%s -- %s%s- %s Nexteer',NxtrConf,char(169),first,last)
      | end
  Vld : Outport
  Prsnt : Outport  Port=2
  wires:
  Constant/1 -> Vld/1
  Previous_Value/1 -> Prsnt/1

== system SF051A_SnsrOffsLrng/SnsrOffsLrng/SnsrOffsLrngPer1/EnableLearning/Perform_TqInpDetn/Enable_PreProcessing/If Action Subsystem ==
  TqInpPrsntRaw : Inport
  Action Port : ActionPort  ActionType=then
  If1 : If  IfExpression=u1
  Merge : Merge
  Merge1 : Merge
  Subsystem5 : Subsystem  Description=|  mask(Copyright Information){none=on}
      | Copyright info block.                                               
      |                                                                     
      | Place copyright information at the top of every subsystem in design.
      mask prompts: none "No parameters"
      mask help: Place copyright information at the top of every subsystem in design.
      mask Display:
      | NxtrConf = 'Nexteer Confidential';
      | 
      | sys = bdroot; %handle for the current model ("system")
      | first = get_param(sys,'Created');
      | first = first(end-3:end);  %year is last four digits
      | 
      | last = get_param(sys,'LastModifiedDate');
      | if isempty(last)
      |     last = datestr(now,'yyyy');
      | else
      |     last = last(end-3:end);
      | end
      | 
      | if strcmp(first,last)
      |     fprintf('%s -- Copyright %s Nexteer',NxtrConf,first)
      | else
      |     fprintf('%s -- %s%s- %s Nexteer',NxtrConf,char(169),first,last)
      | end
  True_False : Subsystem  TreatAsAtomicUnit=on
  True_True : Subsystem  TreatAsAtomicUnit=on
  TqInpPrsntVld : Outport
  TqInpPrsnt : Outport  Port=2
  wires:
  Merge/1 -> TqInpPrsntVld/1
  Merge1/1 -> TqInpPrsnt/1
  True_True/1(Vld) -> Merge/1
  True_False/1(Vld) -> Merge/2
  True_True/2(Prsnt) -> Merge1/1
  True_False/2(Prsnt) -> Merge1/2
  TqInpPrsntRaw/1 -> If1/1
  If1/1 -> True_True/Action
  If1/2 -> True_False/Action

== system SF051A_SnsrOffsLrng/SnsrOffsLrng/SnsrOffsLrngPer1/EnableLearning/Perform_TqInpDetn/Enable_PreProcessing/Preprocessing ==
  note: Runs unconditionally.
  note: Adding two cals at runtime is not efficient, but at
      | least one is likely to be used in online tuning.  Adding
      | them during init would not work for online tuning.
  note: Loop count should = zero when entering this block.
      | Stage 2 block starts execution only after Stage 1 block has been operating for cal1 number of loops.
      | Stage 2 output is only valid once every cal2 number of loops that it has been executing.
  note: Stage 1
  note: Stage 2
  HwTqFild : Inport
  Add : Sum
  Constant : Constant  Value=SnsrOffsLrngTqInpDetnStg1WinSize
  Constant1 : Constant  Value=SnsrOffsLrngTqInpDetnStg2WinSize
  Data Store Write : DataStoreWrite  DataStoreName=TqInpDetnHwTqPreProc
  Data Type Conversion1 : DataTypeConversion  OutDataTypeStr=uint16
  Display1 : DataStoreWrite  DataStoreName=dSnsrOffsLrngTqInpDetnStg1Outp
  Do nothing : Subsystem  TreatAsAtomicUnit=on
  General_Goertzel : Subsystem  TreatAsAtomicUnit=on
  If : If  IfExpression=u1
  If1 : If  IfExpression=u1
  Merge : Merge
  NewOut_ResetCntr : Subsystem  TreatAsAtomicUnit=on
  PrevOut_NoReset : Subsystem  TreatAsAtomicUnit=on
  Relational Operator : RelationalOperator  OutDataTypeStr=boolean
  Relational Operator1 : RelationalOperator  Operator=<  OutDataTypeStr=boolean
  SampleCounter : Subsystem
  Sliding_Goertzel_ver001 : Subsystem
  Subsystem5 : Subsystem  Description=|  mask(Copyright Information){none=on}
      | Copyright info block.                                               
      |                                                                     
      | Place copyright information at the top of every subsystem in design.
      mask prompts: none "No parameters"
      mask help: Place copyright information at the top of every subsystem in design.
      mask Display:
      | NxtrConf = 'Nexteer Confidential';
      | 
      | sys = bdroot; %handle for the current model ("system")
      | first = get_param(sys,'Created');
      | first = first(end-3:end);  %year is last four digits
      | 
      | last = get_param(sys,'LastModifiedDate');
      | if isempty(last)
      |     last = datestr(now,'yyyy');
      | else
      |     last = last(end-3:end);
      | end
      | 
      | if strcmp(first,last)
      |     fprintf('%s -- Copyright %s Nexteer',NxtrConf,first)
      | else
      |     fprintf('%s -- %s%s- %s Nexteer',NxtrConf,char(169),first,last)
      | end
  SampleCntrLim : Outport
  HwTrqPreproc : Outport  Port=2
  wires:
  Sliding_Goertzel_ver001/1(Stg1Outp) -> Display1/1, General_Goertzel/1(Stg1Outp)  "Stg1Outp"
  HwTqFild/1 -> Sliding_Goertzel_ver001/1(HwTqFild)
  If/1 -> General_Goertzel/Action
  General_Goertzel/1(FrqDwnS0) -> NewOut_ResetCntr/1(FrqDwnS0)
  SampleCounter/1(TqInpDetnPreProcEnaLoop) -> Relational Operator/1, [ProcEna], Relational Operator1/1
  Constant1/1 -> Add/1
  If1/2 -> NewOut_ResetCntr/Action
  If1/1 -> PrevOut_NoReset/Action
  PrevOut_NoReset/1(HwTqPreproc) -> Merge/1
  NewOut_ResetCntr/1(HwTqPreproc) -> Merge/2
  Merge/1 -> HwTrqPreproc/1, Data Store Write/1
  General_Goertzel/4(FrqCenS1) -> NewOut_ResetCntr/4(FrqCenS1)
  General_Goertzel/3(FrqCenS0) -> NewOut_ResetCntr/3(FrqCenS0)
  General_Goertzel/6(FrqUpS1) -> NewOut_ResetCntr/6(FrqUpS1)
  General_Goertzel/5(FrqUpS0) -> NewOut_ResetCntr/5(FrqUpS0)
  General_Goertzel/2(FrqDwnS1) -> NewOut_ResetCntr/2(FrqDwnS1)
  Constant/1 -> Data Type Conversion1/1
  Data Type Conversion1/1 -> Relational Operator/2, Add/2
  Add/1 -> SampleCounter/1(HiLim), [CntrLim], SampleCntrLim/1
  Relational Operator/1 -> If/1
  Relational Operator1/1 -> If1/1
  [CntrLim] -> Relational Operator1/2
  If/2 -> Do nothing/Action
  [ProcEna] -> PrevOut_NoReset/1(TqInpDetnPreProcEnaLoop)

== system SF051A_SnsrOffsLrng/SnsrOffsLrng/SnsrOffsLrngPer1/EnableLearning/Perform_TqInpDetn/Enable_PreProcessing/Subsystem5 ==

== system SF051A_SnsrOffsLrng/SnsrOffsLrng/SnsrOffsLrngPer1/EnableLearning/Perform_TqInpDetn/SetStuffToZero/Subsystem5 ==

== system SF051A_SnsrOffsLrng/SnsrOffsLrng/SnsrOffsLrngPer1/Learning/Counter/Increment_SampleCntNeg/Subsystem5 ==

== system SF051A_SnsrOffsLrng/SnsrOffsLrng/SnsrOffsLrngPer1/Learning/Counter/Increment_SampleCntPos/Subsystem5 ==
